simulink model "No_Load_Test"  (R2025a)
settings: Solver=ode23tb  StartTime=0.0  StopTime=5  MaxStep=1e-4  RelTol=1e-3
libraries: spsCurrentMeasurementLib x3, spsACVoltageSourceLib x3, spsVoltageMeasurementLib x3, spsRMSLib x2, spsAsynchronousMachineSIUnitsLib x1, spsMeanLib x1, spsPower3phInstantaneousLib x1, sps_lib x1
settings Model: Creator=Jawad  LastModifiedBy=Jawad

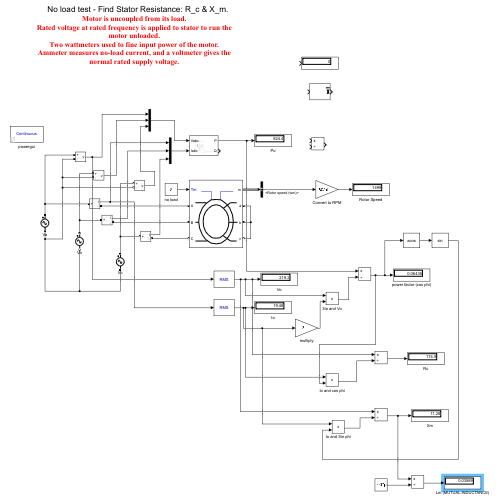
[thumbnail: Simulink's stored preview of the top-level diagram]
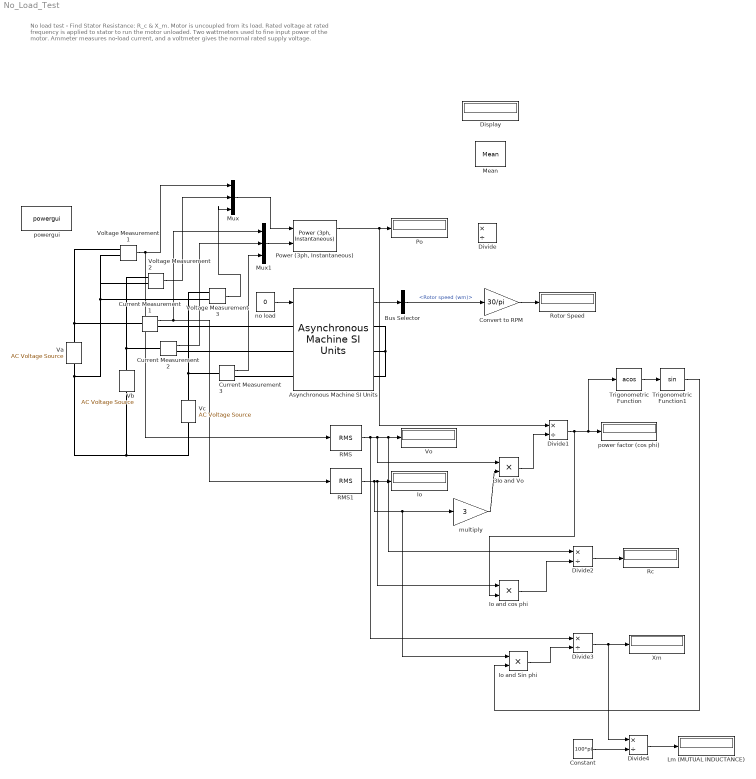
== system No_Load_Test ==
  note: No load test - Find Stator Resistance: R_c & X_m.
      | Motor is uncoupled from its load.
      | Rated voltage at rated frequency is applied to stator to run the motor unloaded.
      | Two wattmeters used to fine input power of the motor.
      | Ammeter measures no-load current, and a voltmeter gives the normal rated supply voltage.
  3Io and Vo : Product
  Asynchronous Machine SI Units : spsAsynchronousMachineSIUnitsLib/Asynchronous Machine SI Units  RotorType=Wound  PresetModel=No  MechanicalLoad=Torque Tm  ShowDetailedParameters=on  ReferenceFrame=Rotor  Units=SI  MeasurementBus=off  NominalParameters=[1.845e+04 460 50]  VoltageRatio=1  Stator=[0.5968 0.0003495]  Rotor=[0.6258 0.005473]  Cage1=[0.4155 0.002066]  Cage2=[0.4168 0.0003495]  Lm=0.0354  Mechanical=[0.05 0.005879 2]  PolePairs=2  InitialConditions=[1 0 0 0 0 0 0 0]  SimulateSaturation=off  Saturation=[14.03593122, 27.81365428, 53.79336849, 72.68890987, 97.98006896, 148.6815601, 215.7428561, 302.9841135, 428.7778367 ; 230, 322, 414, 460, 506, 552, 598, 644, 690]  LoadFlowParameters=1492000  TsPowergui=0  TsBlock=-1  IterativeModel=Trapezoidal non iterative  IterativeDiscreteModel=Trapezoidal non iterative  Pmec=1.492e+006
  Bus Selector : BusSelector  OutputSignals=Mechanical.Rotor speed (wm)
  Constant : Constant  Value=100*pi
  Convert to RPM : Gain  Gain=30/pi
  Current Measurement1 : spsCurrentMeasurementLib/Current Measurement  PhasorSimulation=off  OutputType=Complex  PSBequivalent=0
  Current Measurement2 : spsCurrentMeasurementLib/Current Measurement  PhasorSimulation=off  OutputType=Complex  PSBequivalent=0
  Current Measurement3 : spsCurrentMeasurementLib/Current Measurement  PhasorSimulation=off  OutputType=Complex  PSBequivalent=0
  Display : Display
  Divide{,1..4} (5 alike) : Product  Inputs=*/
  Io : Display
  Io and Sin phi : Product
  Io and cos phi : Product
  Lm (MUTUAL INDUCTANCE) : Display
  Mean : spsMeanLib/Mean  Freq=60  Vinit=0  Ts=0
  Mux : Mux  Inputs=3
  Mux1 : Mux  Inputs=3
  Po : Display
  "Power (3ph, Instantaneous)" : spsPower3phInstantaneousLib/Power (3ph, Instantaneous)
  RMS : spsRMSLib/RMS  TrueRMS=on  Freq=50  RMSInit=0  Ts=0
  RMS1 : spsRMSLib/RMS  TrueRMS=on  Freq=50  RMSInit=0  Ts=0
  Rc : Display
  Rotor Speed : Display
  Trigonometric Function : Trigonometry  Operator=acos
  Trigonometric Function1 : Trigonometry
  Va : spsACVoltageSourceLib/AC Voltage Source  Amplitude=310  Phase=0  Frequency=50  SampleTime=0  Measurements=None  BusType=swing  Pref=10e3  Qref=0  Qmin=-inf  Qmax=+inf
  Vb : spsACVoltageSourceLib/AC Voltage Source  Amplitude=310  Phase=-120  Frequency=50  SampleTime=0  Measurements=None  BusType=swing  Pref=10e3  Qref=0  Qmin=-inf  Qmax=+inf
  Vc : spsACVoltageSourceLib/AC Voltage Source  Amplitude=310  Phase=120  Frequency=50  SampleTime=0  Measurements=None  BusType=swing  Pref=10e3  Qref=0  Qmin=-inf  Qmax=+inf
  Vo : Display
  Voltage Measurement1 : spsVoltageMeasurementLib/Voltage Measurement  PhasorSimulation=off  OutputType=Complex  PSBequivalent=0
  Voltage Measurement2 : spsVoltageMeasurementLib/Voltage Measurement  PhasorSimulation=off  OutputType=Complex  PSBequivalent=0
  Voltage Measurement3 : spsVoltageMeasurementLib/Voltage Measurement  PhasorSimulation=off  OutputType=Complex  PSBequivalent=0
  Xm : Display
  multiply : Gain  Gain=3
  no load : Constant  Value=0
  power factor (cos phi) : Display
  powergui : sps_lib/powergui  Priority=1  SimulationMode=Continuous  SampleTime=50e-6  frequency=60  Iterations=50  frequencyindice=50  Pbase=100e6  ErrMax=1e-4  UnitsV=kV  UnitsW=MW  buscounter=0  FunctionMessages=off  echomessages=off  EnableUseOfTLC=off  CurrentSourceSwitches=off  DisableSnubberDevices=off  DisableRonSwitches=off  DisableVfSwitches=off  DisplayEquations=off  AutomaticDiscreteSolvers=off  SolverType=Tustin/Backward Euler (TBE)  Interpol=off  ExternalGateDelay=off  methode=off  Ts=100  x0status=blocks  SPID=on  SwTol=0  HookPort=off  NonlinearTolerance=1e-4  nMaxIteration=100  ContinueOnMaxIteration=off  RestoreLinks=warning  ResistiveCurrentMeasurement=off  Frange=[0:2:500]  Ylog=off  Xlog=on  ShowGrid=off  save=off  variable=ZData  structure=0  ZoomFFT=off  StartTime=0.0  cycles=1  DisplayStyle=1  fundamental=60  FreqAxis=off  MaxFrequency=1000  frequencyindicesteady=1  RmsSteady=1  display=off
  wires:
  no load/1 -> Asynchronous Machine SI Units/1
  Voltage Measurement1/1 -> RMS/1, Mux/1
  Voltage Measurement2/1 -> Mux/2
  Voltage Measurement3/1 -> Mux/3
  Mux/1 -> "Power (3ph, Instantaneous)"/1
  Mux1/1 -> "Power (3ph, Instantaneous)"/2
  Current Measurement1/1 -> RMS1/1, Mux1/1
  Current Measurement2/1 -> Mux1/2
  Current Measurement3/1 -> Mux1/3
  "Power (3ph, Instantaneous)"/1 -> Divide1/1, Po/1
  RMS/1 -> Divide3/1, 3Io and Vo/1, Divide2/1, Vo/1
  RMS1/1 -> Io and Sin phi/1, multiply/1, Io and cos phi/1, Io/1
  Asynchronous Machine SI Units/1 -> Bus Selector/1
  Bus Selector/1 -> Convert to RPM/1  "<Rotor speed (wm)>"
  Convert to RPM/1 -> Rotor Speed/1
  multiply/1 -> 3Io and Vo/2
  3Io and Vo/1 -> Divide1/2
  Divide1/1 -> Io and cos phi/2, Trigonometric Function/1, power factor (cos phi)/1
  Io and cos phi/1 -> Divide2/2
  Divide2/1 -> Rc/1
  Divide3/1 -> Divide4/1, Xm/1
  Trigonometric Function/1 -> Trigonometric Function1/1
  Trigonometric Function1/1 -> Io and Sin phi/2
  Io and Sin phi/1 -> Divide3/2
  Constant/1 -> Divide4/2
  Divide4/1 -> Lm (MUTUAL INDUCTANCE)/1
  connections:
  Asynchronous Machine SI Units/RConn2 -- Asynchronous Machine SI Units/RConn1 -- Asynchronous Machine SI Units/RConn3
  Va/RConn1 -- Voltage Measurement1/LConn1 -- Current Measurement1/LConn1
  Vb/RConn1 -- Voltage Measurement2/LConn1 -- Current Measurement2/LConn1
  Vc/RConn1 -- Voltage Measurement3/LConn1 -- Current Measurement3/LConn1
  Current Measurement3/RConn1 -- Asynchronous Machine SI Units/LConn3
  Current Measurement2/RConn1 -- Asynchronous Machine SI Units/LConn2
  Current Measurement1/RConn1 -- Asynchronous Machine SI Units/LConn1
  Va/LConn1 -- Voltage Measurement2/LConn2 -- Voltage Measurement1/LConn2 -- Voltage Measurement3/LConn2 -- Vc/LConn1 -- Vb/LConn1
